simulink model "Lab2_AircraftEPS"  (Simulink 8.0)
settings: Solver=ode3  StartTime=0.0  StopTime=10  RelTol=1e-3
PreLoadFcn:
  | warning off
  | Ts=10e-6;
InitFcn:
  | warning off
  | Ts=10e-6;
undefined symbols (not defined in the file or in its folder): D1, Delta, sigbuilder_block
libraries: powerlib x91, sps_avr x4, powerlib_extras x4, checkVoltage x4
(part 1 of 2)
PreSaveFcn:
  | warning on
settings Model: Creator=pidm  LastModifiedBy=forrest  SimulationMode=accelerator
settings SolverCC: AutoInsertRateTranBlk=on
settings DataIOCC: SignalLoggingSaveFormat=ModelDataLogs
settings DebuggingCC: FcnCallInpInsideContextMsg=UseLocalSettings
settings GRTTargetCC: CombineOutputUpdateFcns=off  GRTInterface=on

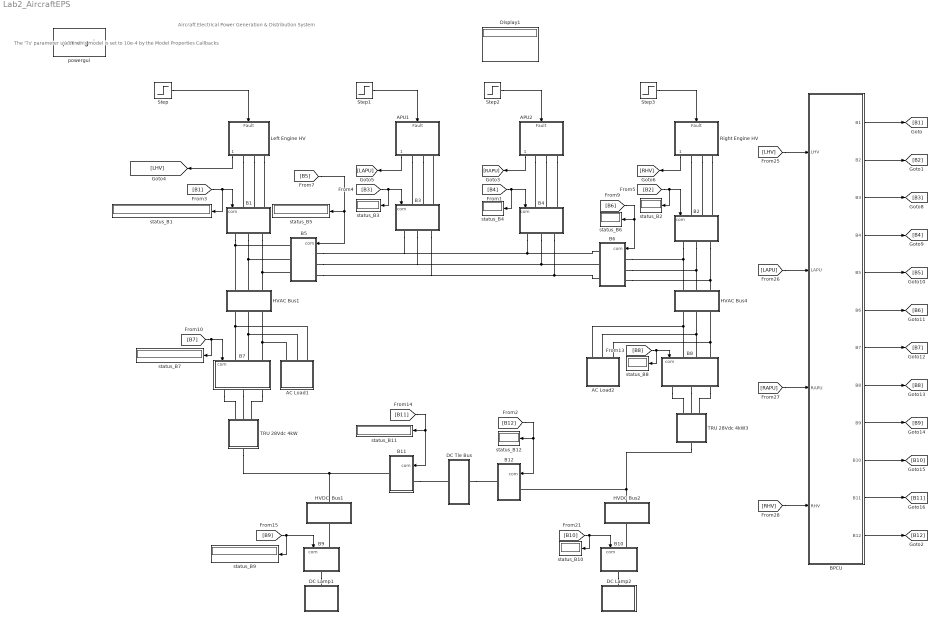
== system Lab2_AircraftEPS ==
  note: The 'Ts' parameter used in this model
      | is set to 10e-4  by the Model Properties Callbacks
  note: Aircraft Electrical Power Generation & Distribution System
  AC Load1 : Subsystem
      mask Display: image(imread('power_aircraft_distribution_ACLamp.jpg','jpg'))
  AC Load2 : Subsystem
      mask Display: image(imread('power_aircraft_distribution_ACLamp.jpg','jpg'))
  APU1 : Subsystem
      mask Display: plot(-80,-50,80,50,[0,9,18,24,29,30,29,24,18,9,0,-9,-18,-24,-29,-30,-29,-24,-18,-9,0],[30,29,24,18,9,0,-9,-18,-24,-29,-30,-29,-24,-18,-9,0,9,18,24,29,30],[-50 -30],[0 0],[50,30],[0 0],[45 35 40 40 40],[15 15 15 20 10],[1 2 3 4 5 6 7 8 9 10 11 12 13 14 15 16 17 18 19 20 21].*1.5-15,[0,9,18,24,29,30,29,24,18,9,0,-9,-18,-24,-29,-30,-29,-24,-18,-9,0]./2.4)
  APU2 : Subsystem
      mask Display: plot(-80,-50,80,50,[0,9,18,24,29,30,29,24,18,9,0,-9,-18,-24,-29,-30,-29,-24,-18,-9,0],[30,29,24,18,9,0,-9,-18,-24,-29,-30,-29,-24,-18,-9,0,9,18,24,29,30],[-50 -30],[0 0],[50,30],[0 0],[45 35 40 40 40],[15 15 15 20 10],[1 2 3 4 5 6 7 8 9 10 11 12 13 14 15 16 17 18 19 20 21].*1.5-15,[0,9,18,24,29,30,29,24,18,9,0,-9,-18,-24,-29,-30,-29,-24,-18,-9,0]./2.4)
  B1 : Subsystem  mask(Contactor){}
      mask help: Simple three phase contactor without a fuse.
      mask Display:
      | plot([0.236212508752942;73.9345152396709], [85.2727156598121;85.2727156598121])
      | patch([0;170.545431319624;170.545431319624;0;0;0.472425017505884;0.472425017505884;170.073006302118;170.073006302118;0.472425017505884;0], [170.545431319624;170.545431319624;0;0;170.545431319624;170.073006302118;0.472425017505884;0.472425017505884;170.073006302118;170.073006302118;170.545431319624], [1;1;1])
      | plot([96.6109160799533;170.309218810871], [85.2727156598121;85.2727156598121])
      | patch([73.9345152396709;79.6036154497415;79.6036154497415;73.9345152396709;73.9345152396709], [119.287316920236;119.287316920236;51.2581143993884;51.2581143993884;119.287316920236], [0;0;0])
      | plot([73.9345152396709;79.6036154497415;79.6036154497415;73.9345152396709;73.9345152396709], [119.287316920236;119.287316920236;51.2581143993884;51.2581143993884;119.287316920236])
      | patch([90.9418158698827;96.6109160799533;96.6109160799533;90.9418158698827;90.9418158698827], [119.287316920236;119.287316920236;51.2581143993884;51.2581143993884;119.287316920236], [0;0;0])
      | plot([90.9418158698827;96.6109160799533;96.6109160799533;90.9418158698827;90.9418158698827], [119.287316920236;119.287316920236;51.2581143993884;51.2581143993884;119.287316920236])
      | ;
  B10 : Subsystem  mask(Contactor){}
      mask help: Simple single phase contactor without a fuse.
      mask Display:
      | plot([0.236212508752942;73.9345152396709], [85.2727156598121;85.2727156598121])
      | patch([0;170.545431319624;170.545431319624;0;0;0.472425017505884;0.472425017505884;170.073006302118;170.073006302118;0.472425017505884;0], [170.545431319624;170.545431319624;0;0;170.545431319624;170.073006302118;0.472425017505884;0.472425017505884;170.073006302118;170.073006302118;170.545431319624], [1;1;1])
      | plot([96.6109160799533;170.309218810871], [85.2727156598121;85.2727156598121])
      | patch([73.9345152396709;79.6036154497415;79.6036154497415;73.9345152396709;73.9345152396709], [119.287316920236;119.287316920236;51.2581143993884;51.2581143993884;119.287316920236], [0;0;0])
      | plot([73.9345152396709;79.6036154497415;79.6036154497415;73.9345152396709;73.9345152396709], [119.287316920236;119.287316920236;51.2581143993884;51.2581143993884;119.287316920236])
      | patch([90.9418158698827;96.6109160799533;96.6109160799533;90.9418158698827;90.9418158698827], [119.287316920236;119.287316920236;51.2581143993884;51.2581143993884;119.287316920236], [0;0;0])
      | plot([90.9418158698827;96.6109160799533;96.6109160799533;90.9418158698827;90.9418158698827], [119.287316920236;119.287316920236;51.2581143993884;51.2581143993884;119.287316920236])
      | ;
  B11 : Subsystem  mask(Contactor){}
      mask help: Simple single phase contactor without a fuse.
      mask Display:
      | plot([0.236212508752942;73.9345152396709], [85.2727156598121;85.2727156598121])
      | patch([0;170.545431319624;170.545431319624;0;0;0.472425017505884;0.472425017505884;170.073006302118;170.073006302118;0.472425017505884;0], [170.545431319624;170.545431319624;0;0;170.545431319624;170.073006302118;0.472425017505884;0.472425017505884;170.073006302118;170.073006302118;170.545431319624], [1;1;1])
      | plot([96.6109160799533;170.309218810871], [85.2727156598121;85.2727156598121])
      | patch([73.9345152396709;79.6036154497415;79.6036154497415;73.9345152396709;73.9345152396709], [119.287316920236;119.287316920236;51.2581143993884;51.2581143993884;119.287316920236], [0;0;0])
      | plot([73.9345152396709;79.6036154497415;79.6036154497415;73.9345152396709;73.9345152396709], [119.287316920236;119.287316920236;51.2581143993884;51.2581143993884;119.287316920236])
      | patch([90.9418158698827;96.6109160799533;96.6109160799533;90.9418158698827;90.9418158698827], [119.287316920236;119.287316920236;51.2581143993884;51.2581143993884;119.287316920236], [0;0;0])
      | plot([90.9418158698827;96.6109160799533;96.6109160799533;90.9418158698827;90.9418158698827], [119.287316920236;119.287316920236;51.2581143993884;51.2581143993884;119.287316920236])
      | ;
  B12 : Subsystem  mask(Contactor){}
      mask help: Simple single phase contactor without a fuse.
      mask Display:
      | plot([0.236212508752942;73.9345152396709], [85.2727156598121;85.2727156598121])
      | patch([0;170.545431319624;170.545431319624;0;0;0.472425017505884;0.472425017505884;170.073006302118;170.073006302118;0.472425017505884;0], [170.545431319624;170.545431319624;0;0;170.545431319624;170.073006302118;0.472425017505884;0.472425017505884;170.073006302118;170.073006302118;170.545431319624], [1;1;1])
      | plot([96.6109160799533;170.309218810871], [85.2727156598121;85.2727156598121])
      | patch([73.9345152396709;79.6036154497415;79.6036154497415;73.9345152396709;73.9345152396709], [119.287316920236;119.287316920236;51.2581143993884;51.2581143993884;119.287316920236], [0;0;0])
      | plot([73.9345152396709;79.6036154497415;79.6036154497415;73.9345152396709;73.9345152396709], [119.287316920236;119.287316920236;51.2581143993884;51.2581143993884;119.287316920236])
      | patch([90.9418158698827;96.6109160799533;96.6109160799533;90.9418158698827;90.9418158698827], [119.287316920236;119.287316920236;51.2581143993884;51.2581143993884;119.287316920236], [0;0;0])
      | plot([90.9418158698827;96.6109160799533;96.6109160799533;90.9418158698827;90.9418158698827], [119.287316920236;119.287316920236;51.2581143993884;51.2581143993884;119.287316920236])
      | ;
  B2 : Subsystem  mask(Contactor){}
      mask help: Simple three phase contactor without a fuse.
      mask Display:
      | plot([0.236212508752942;73.9345152396709], [85.2727156598121;85.2727156598121])
      | patch([0;170.545431319624;170.545431319624;0;0;0.472425017505884;0.472425017505884;170.073006302118;170.073006302118;0.472425017505884;0], [170.545431319624;170.545431319624;0;0;170.545431319624;170.073006302118;0.472425017505884;0.472425017505884;170.073006302118;170.073006302118;170.545431319624], [1;1;1])
      | plot([96.6109160799533;170.309218810871], [85.2727156598121;85.2727156598121])
      | patch([73.9345152396709;79.6036154497415;79.6036154497415;73.9345152396709;73.9345152396709], [119.287316920236;119.287316920236;51.2581143993884;51.2581143993884;119.287316920236], [0;0;0])
      | plot([73.9345152396709;79.6036154497415;79.6036154497415;73.9345152396709;73.9345152396709], [119.287316920236;119.287316920236;51.2581143993884;51.2581143993884;119.287316920236])
      | patch([90.9418158698827;96.6109160799533;96.6109160799533;90.9418158698827;90.9418158698827], [119.287316920236;119.287316920236;51.2581143993884;51.2581143993884;119.287316920236], [0;0;0])
      | plot([90.9418158698827;96.6109160799533;96.6109160799533;90.9418158698827;90.9418158698827], [119.287316920236;119.287316920236;51.2581143993884;51.2581143993884;119.287316920236])
      | ;
  B3 : Subsystem  mask(Contactor){}
      mask help: Simple three phase contactor without a fuse.
      mask Display:
      | plot([0.236212508752942;73.9345152396709], [85.2727156598121;85.2727156598121])
      | patch([0;170.545431319624;170.545431319624;0;0;0.472425017505884;0.472425017505884;170.073006302118;170.073006302118;0.472425017505884;0], [170.545431319624;170.545431319624;0;0;170.545431319624;170.073006302118;0.472425017505884;0.472425017505884;170.073006302118;170.073006302118;170.545431319624], [1;1;1])
      | plot([96.6109160799533;170.309218810871], [85.2727156598121;85.2727156598121])
      | patch([73.9345152396709;79.6036154497415;79.6036154497415;73.9345152396709;73.9345152396709], [119.287316920236;119.287316920236;51.2581143993884;51.2581143993884;119.287316920236], [0;0;0])
      | plot([73.9345152396709;79.6036154497415;79.6036154497415;73.9345152396709;73.9345152396709], [119.287316920236;119.287316920236;51.2581143993884;51.2581143993884;119.287316920236])
      | patch([90.9418158698827;96.6109160799533;96.6109160799533;90.9418158698827;90.9418158698827], [119.287316920236;119.287316920236;51.2581143993884;51.2581143993884;119.287316920236], [0;0;0])
      | plot([90.9418158698827;96.6109160799533;96.6109160799533;90.9418158698827;90.9418158698827], [119.287316920236;119.287316920236;51.2581143993884;51.2581143993884;119.287316920236])
      | ;
  B4 : Subsystem  mask(Contactor){}
      mask help: Simple three phase contactor without a fuse.
      mask Display:
      | plot([0.236212508752942;73.9345152396709], [85.2727156598121;85.2727156598121])
      | patch([0;170.545431319624;170.545431319624;0;0;0.472425017505884;0.472425017505884;170.073006302118;170.073006302118;0.472425017505884;0], [170.545431319624;170.545431319624;0;0;170.545431319624;170.073006302118;0.472425017505884;0.472425017505884;170.073006302118;170.073006302118;170.545431319624], [1;1;1])
      | plot([96.6109160799533;170.309218810871], [85.2727156598121;85.2727156598121])
      | patch([73.9345152396709;79.6036154497415;79.6036154497415;73.9345152396709;73.9345152396709], [119.287316920236;119.287316920236;51.2581143993884;51.2581143993884;119.287316920236], [0;0;0])
      | plot([73.9345152396709;79.6036154497415;79.6036154497415;73.9345152396709;73.9345152396709], [119.287316920236;119.287316920236;51.2581143993884;51.2581143993884;119.287316920236])
      | patch([90.9418158698827;96.6109160799533;96.6109160799533;90.9418158698827;90.9418158698827], [119.287316920236;119.287316920236;51.2581143993884;51.2581143993884;119.287316920236], [0;0;0])
      | plot([90.9418158698827;96.6109160799533;96.6109160799533;90.9418158698827;90.9418158698827], [119.287316920236;119.287316920236;51.2581143993884;51.2581143993884;119.287316920236])
      | ;
  B5 : Subsystem  mask(Contactor){}
      mask help: Simple three phase contactor without a fuse.
      mask Display:
      | plot([0.236212508752942;73.9345152396709], [85.2727156598121;85.2727156598121])
      | patch([0;170.545431319624;170.545431319624;0;0;0.472425017505884;0.472425017505884;170.073006302118;170.073006302118;0.472425017505884;0], [170.545431319624;170.545431319624;0;0;170.545431319624;170.073006302118;0.472425017505884;0.472425017505884;170.073006302118;170.073006302118;170.545431319624], [1;1;1])
      | plot([96.6109160799533;170.309218810871], [85.2727156598121;85.2727156598121])
      | patch([73.9345152396709;79.6036154497415;79.6036154497415;73.9345152396709;73.9345152396709], [119.287316920236;119.287316920236;51.2581143993884;51.2581143993884;119.287316920236], [0;0;0])
      | plot([73.9345152396709;79.6036154497415;79.6036154497415;73.9345152396709;73.9345152396709], [119.287316920236;119.287316920236;51.2581143993884;51.2581143993884;119.287316920236])
      | patch([90.9418158698827;96.6109160799533;96.6109160799533;90.9418158698827;90.9418158698827], [119.287316920236;119.287316920236;51.2581143993884;51.2581143993884;119.287316920236], [0;0;0])
      | plot([90.9418158698827;96.6109160799533;96.6109160799533;90.9418158698827;90.9418158698827], [119.287316920236;119.287316920236;51.2581143993884;51.2581143993884;119.287316920236])
      | ;
  B6 : Subsystem  mask(Contactor){}
      mask help: Simple three phase contactor without a fuse.
      mask Display:
      | plot([0.236212508752942;73.9345152396709], [85.2727156598121;85.2727156598121])
      | patch([0;170.545431319624;170.545431319624;0;0;0.472425017505884;0.472425017505884;170.073006302118;170.073006302118;0.472425017505884;0], [170.545431319624;170.545431319624;0;0;170.545431319624;170.073006302118;0.472425017505884;0.472425017505884;170.073006302118;170.073006302118;170.545431319624], [1;1;1])
      | plot([96.6109160799533;170.309218810871], [85.2727156598121;85.2727156598121])
      | patch([73.9345152396709;79.6036154497415;79.6036154497415;73.9345152396709;73.9345152396709], [119.287316920236;119.287316920236;51.2581143993884;51.2581143993884;119.287316920236], [0;0;0])
      | plot([73.9345152396709;79.6036154497415;79.6036154497415;73.9345152396709;73.9345152396709], [119.287316920236;119.287316920236;51.2581143993884;51.2581143993884;119.287316920236])
      | patch([90.9418158698827;96.6109160799533;96.6109160799533;90.9418158698827;90.9418158698827], [119.287316920236;119.287316920236;51.2581143993884;51.2581143993884;119.287316920236], [0;0;0])
      | plot([90.9418158698827;96.6109160799533;96.6109160799533;90.9418158698827;90.9418158698827], [119.287316920236;119.287316920236;51.2581143993884;51.2581143993884;119.287316920236])
      | ;
  B7 : Subsystem  mask(Contactor){}
      mask help: Simple three phase contactor without a fuse.
      mask Display:
      | plot([0.236212508752942;73.9345152396709], [85.2727156598121;85.2727156598121])
      | patch([0;170.545431319624;170.545431319624;0;0;0.472425017505884;0.472425017505884;170.073006302118;170.073006302118;0.472425017505884;0], [170.545431319624;170.545431319624;0;0;170.545431319624;170.073006302118;0.472425017505884;0.472425017505884;170.073006302118;170.073006302118;170.545431319624], [1;1;1])
      | plot([96.6109160799533;170.309218810871], [85.2727156598121;85.2727156598121])
      | patch([73.9345152396709;79.6036154497415;79.6036154497415;73.9345152396709;73.9345152396709], [119.287316920236;119.287316920236;51.2581143993884;51.2581143993884;119.287316920236], [0;0;0])
      | plot([73.9345152396709;79.6036154497415;79.6036154497415;73.9345152396709;73.9345152396709], [119.287316920236;119.287316920236;51.2581143993884;51.2581143993884;119.287316920236])
      | patch([90.9418158698827;96.6109160799533;96.6109160799533;90.9418158698827;90.9418158698827], [119.287316920236;119.287316920236;51.2581143993884;51.2581143993884;119.287316920236], [0;0;0])
      | plot([90.9418158698827;96.6109160799533;96.6109160799533;90.9418158698827;90.9418158698827], [119.287316920236;119.287316920236;51.2581143993884;51.2581143993884;119.287316920236])
      | ;
  B8 : Subsystem  mask(Contactor){}
      mask help: Simple three phase contactor without a fuse.
      mask Display:
      | plot([0.236212508752942;73.9345152396709], [85.2727156598121;85.2727156598121])
      | patch([0;170.545431319624;170.545431319624;0;0;0.472425017505884;0.472425017505884;170.073006302118;170.073006302118;0.472425017505884;0], [170.545431319624;170.545431319624;0;0;170.545431319624;170.073006302118;0.472425017505884;0.472425017505884;170.073006302118;170.073006302118;170.545431319624], [1;1;1])
      | plot([96.6109160799533;170.309218810871], [85.2727156598121;85.2727156598121])
      | patch([73.9345152396709;79.6036154497415;79.6036154497415;73.9345152396709;73.9345152396709], [119.287316920236;119.287316920236;51.2581143993884;51.2581143993884;119.287316920236], [0;0;0])
      | plot([73.9345152396709;79.6036154497415;79.6036154497415;73.9345152396709;73.9345152396709], [119.287316920236;119.287316920236;51.2581143993884;51.2581143993884;119.287316920236])
      | patch([90.9418158698827;96.6109160799533;96.6109160799533;90.9418158698827;90.9418158698827], [119.287316920236;119.287316920236;51.2581143993884;51.2581143993884;119.287316920236], [0;0;0])
      | plot([90.9418158698827;96.6109160799533;96.6109160799533;90.9418158698827;90.9418158698827], [119.287316920236;119.287316920236;51.2581143993884;51.2581143993884;119.287316920236])
      | ;
  B9 : Subsystem  mask(Contactor){}
      mask help: Simple single phase contactor without a fuse.
      mask Display:
      | plot([0.236212508752942;73.9345152396709], [85.2727156598121;85.2727156598121])
      | patch([0;170.545431319624;170.545431319624;0;0;0.472425017505884;0.472425017505884;170.073006302118;170.073006302118;0.472425017505884;0], [170.545431319624;170.545431319624;0;0;170.545431319624;170.073006302118;0.472425017505884;0.472425017505884;170.073006302118;170.073006302118;170.545431319624], [1;1;1])
      | plot([96.6109160799533;170.309218810871], [85.2727156598121;85.2727156598121])
      | patch([73.9345152396709;79.6036154497415;79.6036154497415;73.9345152396709;73.9345152396709], [119.287316920236;119.287316920236;51.2581143993884;51.2581143993884;119.287316920236], [0;0;0])
      | plot([73.9345152396709;79.6036154497415;79.6036154497415;73.9345152396709;73.9345152396709], [119.287316920236;119.287316920236;51.2581143993884;51.2581143993884;119.287316920236])
      | patch([90.9418158698827;96.6109160799533;96.6109160799533;90.9418158698827;90.9418158698827], [119.287316920236;119.287316920236;51.2581143993884;51.2581143993884;119.287316920236], [0;0;0])
      | plot([90.9418158698827;96.6109160799533;96.6109160799533;90.9418158698827;90.9418158698827], [119.287316920236;119.287316920236;51.2581143993884;51.2581143993884;119.287316920236])
      | ;
  BPCU : Subsystem
  DC Lamp1 : Subsystem
      mask Display: image(imread('power_aircraft_distribution_DCLamp.jpg','jpg'))
  DC Lamp2 : Subsystem
      mask Display: image(imread('power_aircraft_distribution_DCLamp.jpg','jpg'))
  DC Tie Bus : Subsystem
  Display1 : Display
      settings: Floating=on  SampleTime=1e-2
  HVAC Bus1 : Subsystem
  HVAC Bus4 : Subsystem
  HVDC  Bus1 : Subsystem
  HVDC Bus2 : Subsystem
  Left Engine HV : Subsystem
      mask Display: plot(-80,-50,80,50,[0,9,18,24,29,30,29,24,18,9,0,-9,-18,-24,-29,-30,-29,-24,-18,-9,0],[30,29,24,18,9,0,-9,-18,-24,-29,-30,-29,-24,-18,-9,0,9,18,24,29,30],[-50 -30],[0 0],[50,30],[0 0],[45 35 40 40 40],[15 15 15 20 10],[1 2 3 4 5 6 7 8 9 10 11 12 13 14 15 16 17 18 19 20 21].*1.5-15,[0,9,18,24,29,30,29,24,18,9,0,-9,-18,-24,-29,-30,-29,-24,-18,-9,0]./2.4)
  Right Engine HV : Subsystem
      mask Display: plot(-80,-50,80,50,[0,9,18,24,29,30,29,24,18,9,0,-9,-18,-24,-29,-30,-29,-24,-18,-9,0],[30,29,24,18,9,0,-9,-18,-24,-29,-30,-29,-24,-18,-9,0,9,18,24,29,30],[-50 -30],[0 0],[50,30],[0 0],[45 35 40 40 40],[15 15 15 20 10],[1 2 3 4 5 6 7 8 9 10 11 12 13 14 15 16 17 18 19 20 21].*1.5-15,[0,9,18,24,29,30,29,24,18,9,0,-9,-18,-24,-29,-30,-29,-24,-18,-9,0]./2.4)
  Step{,1..3} (4 alike) : Step  SampleTime=0
  TRU 28Vdc 4kW : Subsystem
      mask Display: image(imread('power_aircraft_distribution_TRU.jpg','jpg'))
  TRU 28Vdc 4kW3 : Subsystem
      mask Display: image(imread('power_aircraft_distribution_TRU.jpg','jpg'))
  powergui : powerlib/powergui  SimulationMode=Discrete  SolverType=Tustin  SampleTime=Ts  frequency=60  SPID=off  DisableSnubberDevices=off  DisableRonSwitches=off  DisableVfSwitches=off  SwTol=0  Interpol=off  DisplayEquations=off  FunctionMessages=off  frequencyindice=0  Pbase=100e6  ErrMax=1e-4  Iterations=50  UnitsV=kV  UnitsW=MW  echomessages=off  HookPort=off  EnableUseOfTLC=off  x0status=blocks  RestoreLinks=warning  ResistiveCurrentMeasurement=off  Ylog=off  Xlog=on  ShowGrid=off  save=off  variable=ZData  ZoomFFT=off  StartTime=0.0  cycles=1  DisplayStyle=1  FreqAxis=off  MaxFrequency=1000  frequencyindicesteady=1  display=off  methode=off
  status_B{1..12} (12 alike) : Display
      settings: SampleTime=1e-2
  wires:
  Left Engine HV/1(Vabc) -> [LHV]
  [B1] -> B1/1(com), status_B1/1
  APU1/1(Vabc) -> [LAPU]
  APU2/1(Vabc1) -> [RAPU]
  Right Engine HV/1(Vabc) -> [RHV]
  [B3] -> B3/1(com), status_B3/1
  [B4] -> B4/1(com), status_B4/1
  [B2] -> B2/1(com), status_B2/1
  [B6] -> B6/1(com), status_B6/1
  [B9] -> B9/1(com), status_B9/1
  [LHV] -> BPCU/1(LHV)
  [LAPU] -> BPCU/2(LAPU)
  [RAPU] -> BPCU/3(RAPU)
  [RHV] -> BPCU/4(RHV)
  BPCU/11(B11) -> [B11]
  BPCU/10(B10) -> [B10]
  BPCU/9(B9) -> [B9]
  BPCU/8(B8) -> [B8]
  BPCU/7(B7) -> [B7]
  BPCU/6(B6) -> [B6]
  BPCU/5(B5) -> [B5]
  BPCU/4(B4) -> [B4]
  BPCU/3(B3) -> [B3]
  BPCU/2(B2) -> [B2]
  BPCU/12(B12) -> [B12]
  [B5] -> B5/1(com), status_B5/1
  [B7] -> B7/1(com), status_B7/1
  [B8] -> B8/1(com), status_B8/1
  [B10] -> B10/1(com), status_B10/1
  [B11] -> B11/1(com), status_B11/1
  [B12] -> B12/1(com), status_B12/1
  Step/1 -> Left Engine HV/1(Fault)
  Step1/1 -> APU1/1(Fault)
  Step2/1 -> APU2/1(Fault)
  Step3/1 -> Right Engine HV/1(Fault)
  BPCU/1(B1) -> [B1]
  connections:
  APU2/RConn1 -- B4/LConn1
  APU2/RConn2 -- B4/LConn2
  APU2/RConn3 -- B4/LConn3
  Right Engine HV/RConn1 -- B2/LConn1
  AC Load1/LConn1 -- HVAC Bus1/RConn3 -- B7/LConn3
  AC Load1/LConn2 -- HVAC Bus1/RConn2 -- B7/LConn2
  AC Load1/LConn3 -- HVAC Bus1/RConn1 -- B7/LConn1
  AC Load2/LConn3 -- HVAC Bus4/RConn3 -- B8/LConn3
  AC Load2/LConn1 -- HVAC Bus4/RConn1 -- B8/LConn1
  AC Load2/LConn2 -- HVAC Bus4/RConn2 -- B8/LConn2
  TRU 28Vdc 4kW/RConn1 -- HVDC  Bus1/LConn1 -- B11/RConn1
  TRU 28Vdc 4kW3/RConn1 -- HVDC Bus2/LConn1 -- B12/LConn1
  B9/LConn1 -- HVDC  Bus1/RConn1
  B9/RConn1 -- DC Lamp1/LConn1
  B10/RConn1 -- DC Lamp2/LConn1
  Left Engine HV/RConn1 -- B1/LConn1
  Left Engine HV/RConn2 -- B1/LConn2
  Left Engine HV/RConn3 -- B1/LConn3
  B1/RConn1 -- HVAC Bus1/LConn1 -- B5/RConn1
  B1/RConn2 -- HVAC Bus1/LConn2 -- B5/RConn2
  B1/RConn3 -- HVAC Bus1/LConn3 -- B5/RConn3
  B5/LConn1 -- B3/RConn1 -- B6/RConn1 -- B4/RConn1
  B5/LConn2 -- B3/RConn2 -- B6/RConn2 -- B4/RConn2
  B5/LConn3 -- B3/RConn3 -- B6/RConn3 -- B4/RConn3
  APU1/RConn1 -- B3/LConn1
  APU1/RConn2 -- B3/LConn2
  B3/LConn3 -- APU1/RConn3
  B6/LConn1 -- HVAC Bus4/LConn1 -- B2/RConn1
  B6/LConn2 -- HVAC Bus4/LConn2 -- B2/RConn2
  B6/LConn3 -- HVAC Bus4/LConn3 -- B2/RConn3
  Right Engine HV/RConn2 -- B2/LConn2
  B7/RConn1 -- TRU 28Vdc 4kW/LConn1
  B7/RConn2 -- TRU 28Vdc 4kW/LConn2
  B7/RConn3 -- TRU 28Vdc 4kW/LConn3
  B8/RConn2 -- TRU 28Vdc 4kW3/LConn2
  B8/RConn3 -- TRU 28Vdc 4kW3/LConn3
  B8/RConn1 -- TRU 28Vdc 4kW3/LConn1
  Right Engine HV/RConn3 -- B2/LConn3
  B10/LConn1 -- HVDC Bus2/RConn1
  B11/LConn1 -- DC Tie Bus/RConn1
  DC Tie Bus/LConn1 -- B12/RConn1

== system Lab2_AircraftEPS/AC Load1 ==
  note: AC Load
  Iabc1 : Scope  NumInputPorts=2
      settings: TimeRange=5  YMin=-175~-20  YMax=175~17.5  SaveName=vdc1  SampleTime=10e-6
  Lamp 1000 Watts : powerlib/Elements/Three-Phase Series RLC Load  LConnTagsString=A|B|C  Configuration=Y (grounded)  NominalVoltage=115  NominalFrequency=400  ActivePower=1000  InductivePower=0  CapacitivePower=0  Measurements=None  LoadType=constant Z
  Three Phase  Measurement : powerlib/Measurements/Three-Phase V-I Measurement  VoltageMeasurement=phase-to-phase  SetLabelV=off  LabelV=Vabc  Vpu=off  VpuLL=off  CurrentMeasurement=yes  SetLabelI=off  LabelI=Iabc  Ipu=off  Pbase=100e6  Vbase=500e3  OutputType=Complex  PhasorSimulation=off  PSBequivalent=0
  A : PMIOPort  Port=1  Side=Left
  B : PMIOPort  Port=2  Side=Left
  C : PMIOPort  Port=3  Side=Left
  wires:
  Three Phase  Measurement/1 -> Iabc1/1
  Three Phase  Measurement/2 -> Iabc1/2
  connections:
  Three Phase  Measurement/LConn2 -- B/RConn1
  Three Phase  Measurement/LConn1 -- A/RConn1
  C/RConn1 -- Three Phase  Measurement/LConn3
  Lamp 1000 Watts/LConn1 -- Three Phase  Measurement/RConn1
  Lamp 1000 Watts/LConn2 -- Three Phase  Measurement/RConn2
  Three Phase  Measurement/RConn3 -- Lamp 1000 Watts/LConn3

== system Lab2_AircraftEPS/AC Load2 ==
  note: AC Load
  Iabc1 : Scope  NumInputPorts=2
      settings: TimeRange=5  YMin=-175~-20  YMax=175~17.5  SaveName=vdc3  SampleTime=10e-6
  Lamp 1000 Watts : powerlib/Elements/Three-Phase Series RLC Load  LConnTagsString=A|B|C  Configuration=Y (grounded)  NominalVoltage=115  NominalFrequency=400  ActivePower=1000  InductivePower=0  CapacitivePower=0  Measurements=None  LoadType=constant Z
  Three Phase  Measurement : powerlib/Measurements/Three-Phase V-I Measurement  VoltageMeasurement=phase-to-phase  SetLabelV=off  LabelV=Vabc  Vpu=off  VpuLL=off  CurrentMeasurement=yes  SetLabelI=off  LabelI=Iabc  Ipu=off  Pbase=100e6  Vbase=500e3  OutputType=Complex  PhasorSimulation=off  PSBequivalent=0
  A : PMIOPort  Port=1  Side=Left
  B : PMIOPort  Port=2  Side=Left
  C : PMIOPort  Port=3  Side=Left
  wires:
  Three Phase  Measurement/1 -> Iabc1/1
  Three Phase  Measurement/2 -> Iabc1/2
  connections:
  Three Phase  Measurement/LConn2 -- B/RConn1
  Three Phase  Measurement/LConn1 -- A/RConn1
  C/RConn1 -- Three Phase  Measurement/LConn3
  Lamp 1000 Watts/LConn1 -- Three Phase  Measurement/RConn1
  Lamp 1000 Watts/LConn2 -- Three Phase  Measurement/RConn2
  Three Phase  Measurement/RConn3 -- Lamp 1000 Watts/LConn3

== system Lab2_AircraftEPS/APU1 ==
  Fault : Inport
  Data Type Conversion : DataTypeConversion
  Fault Contactor : Subsystem
  Feedback measurements &  main contactor : Subsystem
  Frequency (Hz) : Display
      settings: SampleTime=1e-2
  Generator  Control Unit (GCU) : Subsystem
      mask Display: image(imread('power_aircraft_distribution_GCU.jpg','jpg'))
  Mechanical engine (turbine) : Subsystem  Tag=STV Subsys  LoadFcn=sigbuilder_block('load');  StartFcn=sigbuilder_block('start');  StopFcn=sigbuilder_block('stop');  ClipboardFcn=sigbuilder_block('clipboard');  mask(Sigbuilder block){}
      mask help: Sigbuilder GUI
      mask init:
      | if ~strcmp(get_param(bdroot(gcbh),'SimulationStatus'),'stopped') tuvar = sigbuilder_block('maskInit'); end
      settings: CopyFcn=sigbuilder_block('copy');  DeleteFcn=sigbuilder_block('delete');  ModelCloseFcn=sigbuilder_block('modelClose');  PreSaveFcn=sigbuilder_block('preSave');  PauseFcn=sigbuilder_block('pause')  ContinueFcn=sigbuilder_block('continue')  NameChangeFcn=sigbuilder_block('namechange');  OpenFcn=sigbuilder_block('open',[274.567 143.773 1029.38 554.126 ]);  CloseFcn=sigbuilder_block('close');
      mask Display: image(imread('power_aircraft_distribution_turbine.jpg','jpg'))
  Power Generation: 50 kVA  synchronous generator : Subsystem
      mask Display: image(imread('power_aircraft_distribution_APU_Generator.jpg','jpg'))
  Sensor : Subsystem
  out_b : PMIOPort  Port=1  Side=Right
  out_c : PMIOPort  Port=2  Side=Right
  out_a : PMIOPort  Port=3  Side=Right
  Vabc : Outport
  wires:
  Feedback measurements &  main contactor/1(Vabc) -> Generator  Control Unit (GCU)/2(voltage sensing)  "Vabc"
  Power Generation: 50 kVA  synchronous generator/1(PMG) -> Generator  Control Unit (GCU)/3(PMG)
  Power Generation: 50 kVA  synchronous generator/2(Out1) -> Frequency (Hz)/1
  Generator  Control Unit (GCU)/2(GLC) -> Data Type Conversion/1
  Feedback measurements &  main contactor/2(Iabc) -> Generator  Control Unit (GCU)/1(current sensing)
  Sensor/1(Vabc) -> Vabc/1
  Data Type Conversion/1 -> Fault Contactor/2(In1)
  Fault/1 -> Fault Contactor/1(Fault)
  Fault Contactor/1(out) -> Feedback measurements &  main contactor/1(GLC control)
  Generator  Control Unit (GCU)/1(Field voltage) -> Power Generation: 50 kVA  synchronous generator/1(fieldvoltage)  "Field"
  Mechanical engine (turbine)/1(Signal 1) -> Power Generation: 50 kVA  synchronous generator/2(Mechanical speed)  "Mechanical Speed"
  connections:
  Power Generation: 50 kVA  synchronous generator/RConn1 -- Feedback measurements &  main contactor/LConn1
  Power Generation: 50 kVA  synchronous generator/RConn2 -- Feedback measurements &  main contactor/LConn2
  Power Generation: 50 kVA  synchronous generator/RConn3 -- Feedback measurements &  main contactor/LConn3
  Feedback measurements &  main contactor/RConn1 -- Sensor/LConn1
  Feedback measurements &  main contactor/RConn2 -- Sensor/LConn2
  Feedback measurements &  main contactor/RConn3 -- Sensor/LConn3
  Sensor/RConn1 -- out_a/RConn1
  Sensor/RConn2 -- out_b/RConn1
  Sensor/RConn3 -- out_c/RConn1

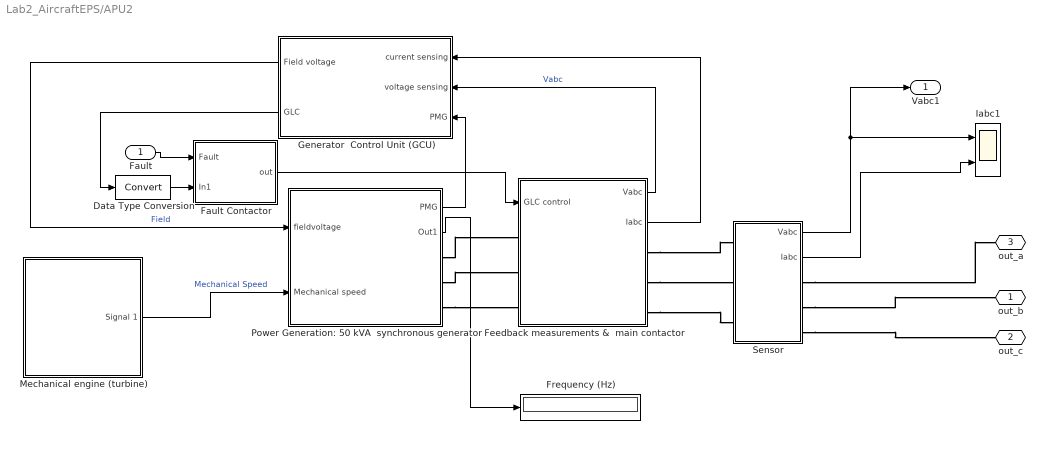
== system Lab2_AircraftEPS/APU2 ==
  Fault : Inport
  Data Type Conversion : DataTypeConversion
  Fault Contactor : Subsystem
  Feedback measurements &  main contactor : Subsystem
  Frequency (Hz) : Display
      settings: SampleTime=1e-2
  Generator  Control Unit (GCU) : Subsystem
      mask Display: image(imread('power_aircraft_distribution_GCU.jpg','jpg'))
  Iabc1 : Scope  NumInputPorts=2
      settings: TimeRange=5  YMin=-8~-300  YMax=8~300  SaveName=vac1  SampleTime=10e-6
  Mechanical engine (turbine) : Subsystem  Tag=STV Subsys  LoadFcn=sigbuilder_block('load');  StartFcn=sigbuilder_block('start');  StopFcn=sigbuilder_block('stop');  ClipboardFcn=sigbuilder_block('clipboard');  mask(Sigbuilder block){}
      mask help: Sigbuilder GUI
      mask init:
      | if ~strcmp(get_param(bdroot(gcbh),'SimulationStatus'),'stopped') tuvar = sigbuilder_block('maskInit'); end
      settings: CopyFcn=sigbuilder_block('copy');  DeleteFcn=sigbuilder_block('delete');  ModelCloseFcn=sigbuilder_block('modelClose');  PreSaveFcn=sigbuilder_block('preSave');  PauseFcn=sigbuilder_block('pause')  ContinueFcn=sigbuilder_block('continue')  NameChangeFcn=sigbuilder_block('namechange');  OpenFcn=sigbuilder_block('open',[339.465 214.661 763.795 427.326 ]);  CloseFcn=sigbuilder_block('close');
      mask Display: image(imread('power_aircraft_distribution_turbine.jpg','jpg'))
  Power Generation: 50 kVA  synchronous generator : Subsystem
      mask Display: image(imread('power_aircraft_distribution_APU_Generator.jpg','jpg'))
  Sensor : Subsystem
  out_b : PMIOPort  Port=1  Side=Right
  out_c : PMIOPort  Port=2  Side=Right
  out_a : PMIOPort  Port=3  Side=Right
  Vabc1 : Outport
  wires:
  Feedback measurements &  main contactor/1(Vabc) -> Generator  Control Unit (GCU)/2(voltage sensing)  "Vabc"
  Power Generation: 50 kVA  synchronous generator/1(PMG) -> Generator  Control Unit (GCU)/3(PMG)
  Power Generation: 50 kVA  synchronous generator/2(Out1) -> Frequency (Hz)/1
  Generator  Control Unit (GCU)/2(GLC) -> Data Type Conversion/1
  Feedback measurements &  main contactor/2(Iabc) -> Generator  Control Unit (GCU)/1(current sensing)
  Sensor/1(Vabc) -> Vabc1/1, Iabc1/1
  Sensor/2(Iabc) -> Iabc1/2
  Data Type Conversion/1 -> Fault Contactor/2(In1)
  Fault/1 -> Fault Contactor/1(Fault)
  Fault Contactor/1(out) -> Feedback measurements &  main contactor/1(GLC control)
  Generator  Control Unit (GCU)/1(Field voltage) -> Power Generation: 50 kVA  synchronous generator/1(fieldvoltage)  "Field"
  Mechanical engine (turbine)/1(Signal 1) -> Power Generation: 50 kVA  synchronous generator/2(Mechanical speed)  "Mechanical Speed"
  connections:
  Power Generation: 50 kVA  synchronous generator/RConn1 -- Feedback measurements &  main contactor/LConn1
  Power Generation: 50 kVA  synchronous generator/RConn2 -- Feedback measurements &  main contactor/LConn2
  Power Generation: 50 kVA  synchronous generator/RConn3 -- Feedback measurements &  main contactor/LConn3
  Feedback measurements &  main contactor/RConn1 -- Sensor/LConn1
  Feedback measurements &  main contactor/RConn2 -- Sensor/LConn2
  Feedback measurements &  main contactor/RConn3 -- Sensor/LConn3
  Sensor/RConn1 -- out_a/RConn1
  Sensor/RConn2 -- out_b/RConn1
  Sensor/RConn3 -- out_c/RConn1

== system Lab2_AircraftEPS/B1 ==
  com : Inport
  Contactor : Subsystem
  A1 : PMIOPort  Port=1  Side=Right
  B1 : PMIOPort  Port=2  Side=Right
  C1 : PMIOPort  Port=3  Side=Right
  A : PMIOPort  Port=4  Side=Left
  B : PMIOPort  Port=5  Side=Left
  C : PMIOPort  Port=6  Side=Left
  wires:
  com/1 -> Contactor/1(com)
  connections:
  Contactor/RConn1 -- A1/RConn1
  Contactor/RConn2 -- B1/RConn1
  Contactor/RConn3 -- C1/RConn1
  A/RConn1 -- Contactor/LConn1
  B/RConn1 -- Contactor/LConn2
  C/RConn1 -- Contactor/LConn3

== system Lab2_AircraftEPS/B10 ==
  com : Inport
  Contactor : Subsystem
  A1 : PMIOPort  Port=1  Side=Right
  A : PMIOPort  Port=2  Side=Left
  wires:
  com/1 -> Contactor/1(com)
  connections:
  Contactor/RConn1 -- A1/RConn1
  A/RConn1 -- Contactor/LConn1

== system Lab2_AircraftEPS/B11 ==
  com : Inport
  Contactor : Subsystem
  A1 : PMIOPort  Port=1  Side=Right
  A : PMIOPort  Port=2  Side=Left
  wires:
  com/1 -> Contactor/1(com)
  connections:
  Contactor/RConn1 -- A1/RConn1
  A/RConn1 -- Contactor/LConn1

== system Lab2_AircraftEPS/B12 ==
  com : Inport
  Contactor : Subsystem
  A1 : PMIOPort  Port=1  Side=Right
  A : PMIOPort  Port=2  Side=Left
  wires:
  com/1 -> Contactor/1(com)
  connections:
  Contactor/RConn1 -- A1/RConn1
  A/RConn1 -- Contactor/LConn1

== system Lab2_AircraftEPS/B2 ==
  com : Inport
  Contactor : Subsystem
  A1 : PMIOPort  Port=1  Side=Right
  B1 : PMIOPort  Port=2  Side=Right
  C1 : PMIOPort  Port=3  Side=Right
  A : PMIOPort  Port=4  Side=Left
  B : PMIOPort  Port=5  Side=Left
  C : PMIOPort  Port=6  Side=Left
  wires:
  com/1 -> Contactor/1(com)
  connections:
  Contactor/RConn1 -- A1/RConn1
  Contactor/RConn2 -- B1/RConn1
  Contactor/RConn3 -- C1/RConn1
  A/RConn1 -- Contactor/LConn1
  B/RConn1 -- Contactor/LConn2
  C/RConn1 -- Contactor/LConn3

== system Lab2_AircraftEPS/B3 ==
  com : Inport
  Contactor : Subsystem
  A1 : PMIOPort  Port=1  Side=Right
  B1 : PMIOPort  Port=2  Side=Right
  C1 : PMIOPort  Port=3  Side=Right
  A : PMIOPort  Port=4  Side=Left
  B : PMIOPort  Port=5  Side=Left
  C : PMIOPort  Port=6  Side=Left
  wires:
  com/1 -> Contactor/1(com)
  connections:
  Contactor/RConn1 -- A1/RConn1
  Contactor/RConn2 -- B1/RConn1
  Contactor/RConn3 -- C1/RConn1
  A/RConn1 -- Contactor/LConn1
  B/RConn1 -- Contactor/LConn2
  C/RConn1 -- Contactor/LConn3

== system Lab2_AircraftEPS/B4 ==
  com : Inport
  Contactor : Subsystem
  A1 : PMIOPort  Port=1  Side=Right
  B1 : PMIOPort  Port=2  Side=Right
  C1 : PMIOPort  Port=3  Side=Right
  A : PMIOPort  Port=4  Side=Left
  B : PMIOPort  Port=5  Side=Left
  C : PMIOPort  Port=6  Side=Left
  wires:
  com/1 -> Contactor/1(com)
  connections:
  Contactor/RConn1 -- A1/RConn1
  Contactor/RConn2 -- B1/RConn1
  Contactor/RConn3 -- C1/RConn1
  A/RConn1 -- Contactor/LConn1
  B/RConn1 -- Contactor/LConn2
  C/RConn1 -- Contactor/LConn3

== system Lab2_AircraftEPS/B5 ==
  com : Inport
  Contactor : Subsystem
  A1 : PMIOPort  Port=1  Side=Right
  B1 : PMIOPort  Port=2  Side=Right
  C1 : PMIOPort  Port=3  Side=Right
  A : PMIOPort  Port=4  Side=Left
  B : PMIOPort  Port=5  Side=Left
  C : PMIOPort  Port=6  Side=Left
  wires:
  com/1 -> Contactor/1(com)
  connections:
  Contactor/RConn1 -- A1/RConn1
  Contactor/RConn2 -- B1/RConn1
  Contactor/RConn3 -- C1/RConn1
  A/RConn1 -- Contactor/LConn1
  B/RConn1 -- Contactor/LConn2
  C/RConn1 -- Contactor/LConn3

== system Lab2_AircraftEPS/B6 ==
  com : Inport
  Contactor : Subsystem
  A1 : PMIOPort  Port=1  Side=Right
  B1 : PMIOPort  Port=2  Side=Right
  C1 : PMIOPort  Port=3  Side=Right
  A : PMIOPort  Port=4  Side=Left
  B : PMIOPort  Port=5  Side=Left
  C : PMIOPort  Port=6  Side=Left
  wires:
  com/1 -> Contactor/1(com)
  connections:
  Contactor/RConn1 -- A1/RConn1
  Contactor/RConn2 -- B1/RConn1
  Contactor/RConn3 -- C1/RConn1
  A/RConn1 -- Contactor/LConn1
  B/RConn1 -- Contactor/LConn2
  C/RConn1 -- Contactor/LConn3

== system Lab2_AircraftEPS/B7 ==
  com : Inport
  Contactor : Subsystem
  A1 : PMIOPort  Port=1  Side=Right
  B1 : PMIOPort  Port=2  Side=Right
  C1 : PMIOPort  Port=3  Side=Right
  A : PMIOPort  Port=4  Side=Left
  B : PMIOPort  Port=5  Side=Left
  C : PMIOPort  Port=6  Side=Left
  wires:
  com/1 -> Contactor/1(com)
  connections:
  Contactor/RConn1 -- A1/RConn1
  Contactor/RConn2 -- B1/RConn1
  Contactor/RConn3 -- C1/RConn1
  A/RConn1 -- Contactor/LConn1
  B/RConn1 -- Contactor/LConn2
  C/RConn1 -- Contactor/LConn3

== system Lab2_AircraftEPS/B8 ==
  com : Inport
  Contactor : Subsystem
  A1 : PMIOPort  Port=1  Side=Right
  B1 : PMIOPort  Port=2  Side=Right
  C1 : PMIOPort  Port=3  Side=Right
  A : PMIOPort  Port=4  Side=Left
  B : PMIOPort  Port=5  Side=Left
  C : PMIOPort  Port=6  Side=Left
  wires:
  com/1 -> Contactor/1(com)
  connections:
  Contactor/RConn1 -- A1/RConn1
  Contactor/RConn2 -- B1/RConn1
  Contactor/RConn3 -- C1/RConn1
  A/RConn1 -- Contactor/LConn1
  B/RConn1 -- Contactor/LConn2
  C/RConn1 -- Contactor/LConn3

== system Lab2_AircraftEPS/B9 ==
  com : Inport
  Contactor : Subsystem
  A1 : PMIOPort  Port=1  Side=Right
  A : PMIOPort  Port=2  Side=Left
  wires:
  com/1 -> Contactor/1(com)
  connections:
  Contactor/RConn1 -- A1/RConn1
  A/RConn1 -- Contactor/LConn1

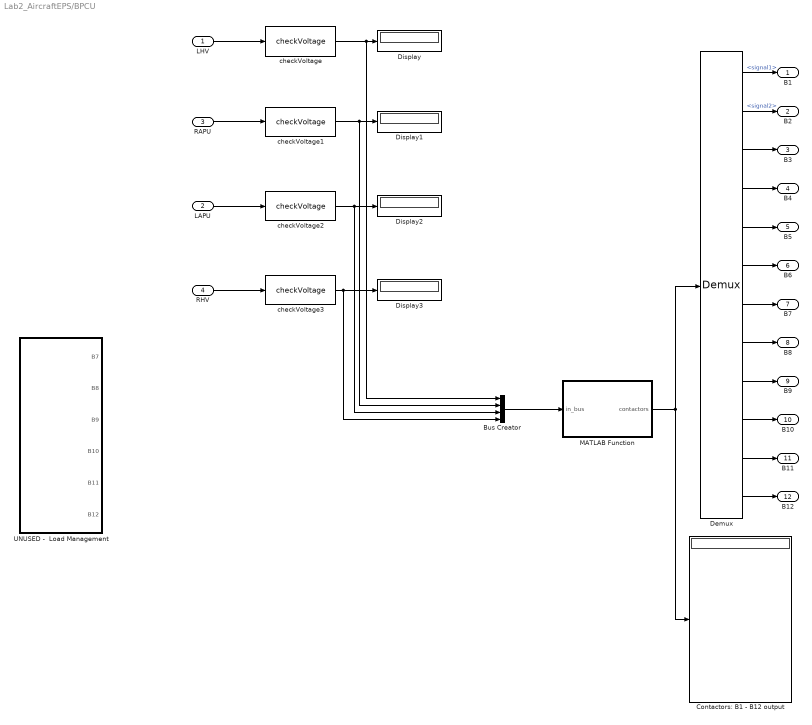
== system Lab2_AircraftEPS/BPCU ==
  LHV : Inport
  LAPU : Inport  Port=2
  RAPU : Inport  Port=3
  RHV : Inport  Port=4
  Bus Creator : BusCreator
  Contactors: B1 - B12 output : Display
  Demux : Demux  Outputs=12
  Display{,1..3} (4 alike) : Display
  MATLAB Function : MATLAB Function  TreatAsAtomicUnit=on
  UNUSED -  Load Management : Subsystem
  checkVoltage{,1..3} (4 alike) : checkVoltage/checkVoltage
  B1 : Outport
  B2 : Outport  Port=2
  B3 : Outport  Port=3
  B4 : Outport  Port=4
  B5 : Outport  Port=5
  B6 : Outport  Port=6
  B7 : Outport  Port=7
  B8 : Outport  Port=8
  B9 : Outport  Port=9
  B10 : Outport  Port=10
  B11 : Outport  Port=11
  B12 : Outport  Port=12
  wires:
  LHV/1 -> checkVoltage/1
  checkVoltage/1 -> Bus Creator/1, Display/1
  RAPU/1 -> checkVoltage1/1
  checkVoltage1/1 -> Bus Creator/2, Display1/1
  LAPU/1 -> checkVoltage2/1
  RHV/1 -> checkVoltage3/1
  checkVoltage3/1 -> Bus Creator/4, Display3/1
  checkVoltage2/1 -> Bus Creator/3, Display2/1
  Bus Creator/1 -> MATLAB Function/1(in_bus)
  MATLAB Function/1(contactors) -> Contactors: B1 - B12 output/1, Demux/1
  Demux/1 -> B1/1  "<signal1>"
  Demux/2 -> B2/1  "<signal2>"
  Demux/3 -> B3/1
  Demux/4 -> B4/1
  Demux/5 -> B5/1
  Demux/6 -> B6/1
  Demux/7 -> B7/1
  Demux/8 -> B8/1
  Demux/9 -> B9/1
  Demux/10 -> B10/1
  Demux/11 -> B11/1
  Demux/12 -> B12/1

== system Lab2_AircraftEPS/DC Lamp1 ==
  note: DC Load
  Current Measurement : powerlib/Measurements/Current Measurement  PhasorSimulation=off  OutputType=Complex  PSBequivalent=0
  Ground1 : powerlib/Elements/Ground  LConnTagsString=a
  Iabc1 : Scope  NumInputPorts=2
      settings: TimeRange=5  YMin=-2.5~-2.5  YMax=30~30  SaveName=vdc  SampleTime=10e-6
  Series RLC Branch3 : powerlib/Elements/Series RLC Branch  LConnTagsString=__new0  RConnTagsString=__new0  BranchType=R  Resistance=1  Inductance=[]  SetiL0=off  InitialCurrent=0  Capacitance=[]  Setx0=off  InitialVoltage=0  Measurements=Branch voltage and current
  Voltage Measurement : powerlib/Measurements/Voltage Measurement  PhasorSimulation=off  OutputType=Complex  PSBequivalent=0
  + : PMIOPort  Port=1  Side=Left
  wires:
  Current Measurement/1 -> Iabc1/1
  Voltage Measurement/1 -> Iabc1/2
  connections:
  Voltage Measurement/LConn2 -- Series RLC Branch3/RConn1 -- Ground1/LConn1
  Voltage Measurement/LConn1 -- +/RConn1 -- Current Measurement/LConn1
  Current Measurement/RConn1 -- Series RLC Branch3/LConn1

== system Lab2_AircraftEPS/DC Lamp2 ==
  note: DC Load
  Current Measurement : powerlib/Measurements/Current Measurement  PhasorSimulation=off  OutputType=Complex  PSBequivalent=0
  Ground2 : powerlib/Elements/Ground  LConnTagsString=a
  Iabc1 : Scope  NumInputPorts=2
      settings: TimeRange=5  YMin=-2.5~-2.5  YMax=30~30  SaveName=vdc2  SampleTime=10e-6
  Series RLC Branch3 : powerlib/Elements/Series RLC Branch  LConnTagsString=__new0  RConnTagsString=__new0  BranchType=R  Resistance=1  Inductance=[]  SetiL0=off  InitialCurrent=0  Capacitance=[]  Setx0=off  InitialVoltage=0  Measurements=Branch voltage and current
  Voltage Measurement : powerlib/Measurements/Voltage Measurement  PhasorSimulation=off  OutputType=Complex  PSBequivalent=0
  + : PMIOPort  Port=1  Side=Left
  wires:
  Current Measurement/1 -> Iabc1/1
  Voltage Measurement/1 -> Iabc1/2
  connections:
  Voltage Measurement/LConn2 -- Series RLC Branch3/RConn1 -- Ground2/LConn1
  Voltage Measurement/LConn1 -- +/RConn1 -- Current Measurement/LConn1
  Current Measurement/RConn1 -- Series RLC Branch3/LConn1

== system Lab2_AircraftEPS/DC Tie Bus ==
  a : PMIOPort  Port=1  Side=Left
  "a " : PMIOPort  Port=2  Side=Right
  connections:
  a/RConn1 -- "a "/RConn1

== system Lab2_AircraftEPS/HVAC Bus1 ==
  a : PMIOPort  Port=1  Side=Left
  b : PMIOPort  Port=2  Side=Left
  c : PMIOPort  Port=3  Side=Left
  "a " : PMIOPort  Port=4  Side=Right
  "b " : PMIOPort  Port=5  Side=Right
  "c " : PMIOPort  Port=6  Side=Right
  connections:
  b/RConn1 -- "b "/RConn1
  c/RConn1 -- "c "/RConn1
  a/RConn1 -- "a "/RConn1

== system Lab2_AircraftEPS/HVAC Bus4 ==
  a : PMIOPort  Port=1  Side=Left
  b : PMIOPort  Port=2  Side=Left
  c : PMIOPort  Port=3  Side=Left
  "a " : PMIOPort  Port=4  Side=Right
  "b " : PMIOPort  Port=5  Side=Right
  "c " : PMIOPort  Port=6  Side=Right
  connections:
  b/RConn1 -- "b "/RConn1
  c/RConn1 -- "c "/RConn1
  a/RConn1 -- "a "/RConn1

== system Lab2_AircraftEPS/HVDC  Bus1 ==
  a : PMIOPort  Port=1  Side=Left
  "a " : PMIOPort  Port=2  Side=Right
  connections:
  a/RConn1 -- "a "/RConn1

== system Lab2_AircraftEPS/HVDC Bus2 ==
  a : PMIOPort  Port=1  Side=Left
  "a " : PMIOPort  Port=2  Side=Right
  connections:
  a/RConn1 -- "a "/RConn1

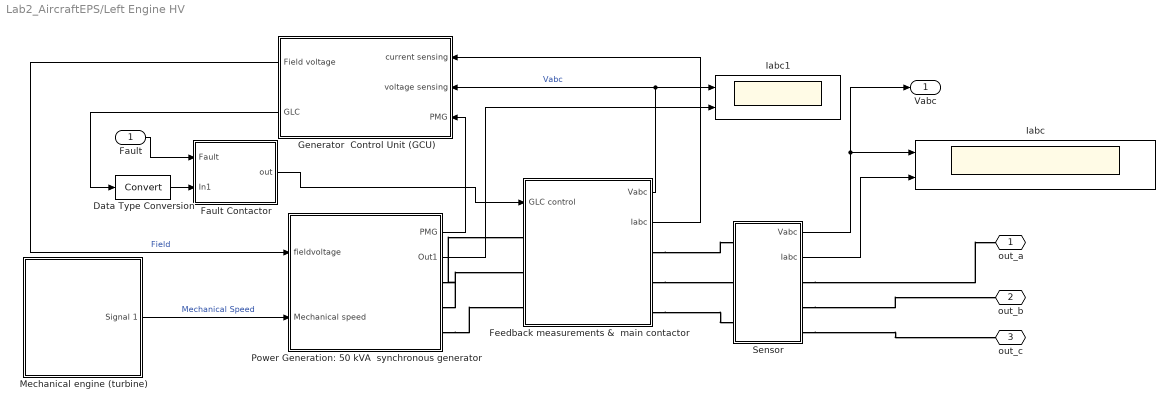
== system Lab2_AircraftEPS/Left Engine HV ==
  Fault : Inport
  Data Type Conversion : DataTypeConversion
  Fault Contactor : Subsystem
  Feedback measurements &  main contactor : Subsystem
  Generator  Control Unit (GCU) : Subsystem
      mask Display: image(imread('power_aircraft_distribution_GCU.jpg','jpg'))
  Iabc : Scope  NumInputPorts=2
      settings: TimeRange=5  YMin=-175~-20  YMax=175~20  SaveName=vac  SampleTime=10e-6
  Iabc1 : Scope  NumInputPorts=2
      settings: TimeRange=5  YMin=-250~260  YMax=250~400  SaveName=vac2  SampleTime=10e-6
  Mechanical engine (turbine) : Subsystem  Tag=STV Subsys  LoadFcn=sigbuilder_block('load');  StartFcn=sigbuilder_block('start');  StopFcn=sigbuilder_block('stop');  ClipboardFcn=sigbuilder_block('clipboard');  mask(Sigbuilder block){}
      mask help: Sigbuilder GUI
      mask init:
      | if ~strcmp(get_param(bdroot(gcbh),'SimulationStatus'),'stopped') tuvar = sigbuilder_block('maskInit'); end
      settings: CopyFcn=sigbuilder_block('copy');  DeleteFcn=sigbuilder_block('delete');  ModelCloseFcn=sigbuilder_block('modelClose');  PreSaveFcn=sigbuilder_block('preSave');  PauseFcn=sigbuilder_block('pause')  ContinueFcn=sigbuilder_block('continue')  NameChangeFcn=sigbuilder_block('namechange');  OpenFcn=sigbuilder_block('open',[323.25 315.75 528 359.25 ]);  CloseFcn=sigbuilder_block('close');
      mask Display: image(imread('power_aircraft_distribution_turbine.jpg','jpg'))
  Power Generation: 50 kVA  synchronous generator : Subsystem
      mask Display: image(imread('power_aircraft_distribution_APU_Generator.jpg','jpg'))
  Sensor : Subsystem
  out_a : PMIOPort  Port=1  Side=Right
  out_b : PMIOPort  Port=2  Side=Right
  out_c : PMIOPort  Port=3  Side=Right
  Vabc : Outport
  wires:
  Feedback measurements &  main contactor/1(Vabc) -> Generator  Control Unit (GCU)/2(voltage sensing), Iabc1/1  "Vabc"
  Power Generation: 50 kVA  synchronous generator/1(PMG) -> Generator  Control Unit (GCU)/3(PMG)
  Power Generation: 50 kVA  synchronous generator/2(Out1) -> Iabc1/2
  Feedback measurements &  main contactor/2(Iabc) -> Generator  Control Unit (GCU)/1(current sensing)
  Sensor/1(Vabc) -> Vabc/1, Iabc/1
  Sensor/2(Iabc) -> Iabc/2
  Data Type Conversion/1 -> Fault Contactor/2(In1)
  Fault/1 -> Fault Contactor/1(Fault)
  Generator  Control Unit (GCU)/1(Field voltage) -> Power Generation: 50 kVA  synchronous generator/1(fieldvoltage)  "Field"
  Mechanical engine (turbine)/1(Signal 1) -> Power Generation: 50 kVA  synchronous generator/2(Mechanical speed)  "Mechanical Speed"
  Generator  Control Unit (GCU)/2(GLC) -> Data Type Conversion/1
  Fault Contactor/1(out) -> Feedback measurements &  main contactor/1(GLC control)
  connections:
  Power Generation: 50 kVA  synchronous generator/RConn1 -- Feedback measurements &  main contactor/LConn1
  Power Generation: 50 kVA  synchronous generator/RConn2 -- Feedback measurements &  main contactor/LConn2
  Power Generation: 50 kVA  synchronous generator/RConn3 -- Feedback measurements &  main contactor/LConn3
  Feedback measurements &  main contactor/RConn1 -- Sensor/LConn1
  Feedback measurements &  main contactor/RConn2 -- Sensor/LConn2
  Feedback measurements &  main contactor/RConn3 -- Sensor/LConn3
  Sensor/RConn1 -- out_a/RConn1
  Sensor/RConn2 -- out_b/RConn1
  Sensor/RConn3 -- out_c/RConn1

== system Lab2_AircraftEPS/Right Engine HV ==
  Fault : Inport
  Data Type Conversion : DataTypeConversion
  Fault Contactor : Subsystem
  Feedback measurements &  main contactor : Subsystem
  Frequency (Hz) : Display
      settings: SampleTime=1e-2
  Generator  Control Unit (GCU) : Subsystem
      mask Display: image(imread('power_aircraft_distribution_GCU.jpg','jpg'))
  Mechanical engine (turbine) : Subsystem  Tag=STV Subsys  LoadFcn=sigbuilder_block('load');  StartFcn=sigbuilder_block('start');  StopFcn=sigbuilder_block('stop');  ClipboardFcn=sigbuilder_block('clipboard');  mask(Sigbuilder block){}
      mask help: Sigbuilder GUI
      mask init:
      | if ~strcmp(get_param(bdroot(gcbh),'SimulationStatus'),'stopped') tuvar = sigbuilder_block('maskInit'); end
      settings: CopyFcn=sigbuilder_block('copy');  DeleteFcn=sigbuilder_block('delete');  ModelCloseFcn=sigbuilder_block('modelClose');  PreSaveFcn=sigbuilder_block('preSave');  PauseFcn=sigbuilder_block('pause')  ContinueFcn=sigbuilder_block('continue')  NameChangeFcn=sigbuilder_block('namechange');  OpenFcn=sigbuilder_block('open',[361.43 20.9669 788.756 420.337 ]);  CloseFcn=sigbuilder_block('close');
      mask Display: image(imread('power_aircraft_distribution_turbine.jpg','jpg'))
  Power Generation: 50 kVA  synchronous generator : Subsystem
      mask Display: image(imread('power_aircraft_distribution_APU_Generator.jpg','jpg'))
  Sensor : Subsystem
  out_b : PMIOPort  Port=1  Side=Right
  out_c : PMIOPort  Port=2  Side=Right
  out_a : PMIOPort  Port=3  Side=Right
  Vabc : Outport
  wires:
  Feedback measurements &  main contactor/1(Vabc) -> Generator  Control Unit (GCU)/2(voltage sensing)  "Vabc"
  Power Generation: 50 kVA  synchronous generator/1(PMG) -> Generator  Control Unit (GCU)/3(PMG)
  Power Generation: 50 kVA  synchronous generator/2(Out1) -> Frequency (Hz)/1
  Generator  Control Unit (GCU)/2(GLC) -> Data Type Conversion/1
  Feedback measurements &  main contactor/2(Iabc) -> Generator  Control Unit (GCU)/1(current sensing)
  Sensor/1(Vabc) -> Vabc/1
  Data Type Conversion/1 -> Fault Contactor/2(In1)
  Fault/1 -> Fault Contactor/1(Fault)
  Fault Contactor/1(out) -> Feedback measurements &  main contactor/1(GLC control)
  Generator  Control Unit (GCU)/1(Field voltage) -> Power Generation: 50 kVA  synchronous generator/1(fieldvoltage)  "Field"
  Mechanical engine (turbine)/1(Signal 1) -> Power Generation: 50 kVA  synchronous generator/2(Mechanical speed)  "Mechanical Speed"
  connections:
  Power Generation: 50 kVA  synchronous generator/RConn1 -- Feedback measurements &  main contactor/LConn1
  Power Generation: 50 kVA  synchronous generator/RConn2 -- Feedback measurements &  main contactor/LConn2
  Power Generation: 50 kVA  synchronous generator/RConn3 -- Feedback measurements &  main contactor/LConn3
  Feedback measurements &  main contactor/RConn1 -- Sensor/LConn1
  Feedback measurements &  main contactor/RConn2 -- Sensor/LConn2
  Feedback measurements &  main contactor/RConn3 -- Sensor/LConn3
  Sensor/RConn1 -- out_a/RConn1
  Sensor/RConn2 -- out_b/RConn1
  Sensor/RConn3 -- out_c/RConn1
